simulink model "panda"  (R2022b)
settings: Solver=VariableStepAuto  StartTime=0.0  StopTime=10  EnableMultiTasking=on
values from neighbouring files (symbols this model uses):
  en = 1    [main_manipulator.m]
  q0 = [-pi/4 -3*pi/4]    [main_manipulator.m]
  q2 = [-0.785398163397 -0.78574787628 -0.786097014423 -0.786445577071 -0.786793563474 -0.787140972883 -0.787487804552 -0.787834057739 -0.788179731704 -0.788524825712 -0.78886933903 -0.789213270926 ... (6284 elements, 1x6284)]    [q2.mat]
  sr = 0.01    [main_manipulator.m]
  T = 1    [main_manipulator.m]
  w0 = 0.*[(q2(2)-q2(1))/(T/length(q2)) (q4(2)-q4(1))/(T/length(q4))]    [main_manipulator.m]
undefined symbols (not defined in the file or in its folder): Acceleration_1, Acceleration_2, Center_1, Center_2, magnitude, Pitch_1, Pitch_2, q4, Radius_1, Radius_2, Transformation_1, Transformation_2, tt, X, x_ee, Y, y_ee, Z
libraries: nesl_utility x15, sm_lib x14, simulink x14, slpidlib x4, franka_simulink_library x2, rllib x1
(part 1 of 2)
settings Model: Creator=Metti  LastModifiedBy=s2ajami
settings SolverCC: ZeroCrossControl=DisableAll
settings DataIOCC: LimitDataPoints=on  SaveFormat=Array  ReturnWorkspaceOutputs=off
settings OptimizationCC: ExpressionDepthLimit=2147483647  LifeSpan=inf
settings DebuggingCC: UnderspecifiedInitializationDetection=Classic  MergeDetectMultiDrivingBlocksExec=none  SolverPrmCheckMsg=warning  MultiTaskDSMMsg=warning  MultiTaskCondExecSysMsg=none  FcnCallInpInsideContextMsg=warning  UnconnectedInputMsg=warning  UnconnectedOutputMsg=warning  UnconnectedLineMsg=warning  StateNameClashWarn=warning  SFUnexpectedBacktrackingDiag=warning  SFNoUnconditionalDefaultTransitionDiag=warning  SFExecutionAtInitializationDiag=none  SFMachineParentedDataDiag=warning  ArithmeticOperatorsInVariantConditions=warning
settings HardwareCC: ProdBitPerPointer=32  ProdBitPerSizeT=32  ProdBitPerPtrDiffT=32  ProdLargestAtomicFloat=None  ProdIntDivRoundTo=Undefined  ProdEndianess=Unspecified  ProdWordSize=32  ProdHWDeviceType=32-bit Generic
settings ModelReferenceCC: EnableRefExpFcnMdlSchedulingChecks=on  PropagateSignalLabelsOutOfModel=off
settings SFSimCC: SimUseLocalCustomCode=off  CustomCodeUndefinedFunction=UseInterfaceOnly
settings RTWCC: RTWUseLocalCustomCode=off
settings CodeAppCC: StateflowObjectComments=on
settings GRTTargetCC: TargetLangStandard=C89/C90 (ANSI)
settings ConfigComp: CovMetricSettings=dw  CovSaveCumulativeToWorkspaceVar=on  CovSaveSingleToWorkspaceVar=on  CovExternalEMLEnable=off
settings SimscapeCC: SimscapeNormalizeSystem=off
settings ConfigurationSet: Description=SimMechanics 2G
settings ExplorerConfigSet: InternalSimMechanicsExplorerSettings="<ExplorerConfiguration><canonicalview>default</canonicalview><TilePanel><TileInfo><Tiles Columns=\"1\" Count=\"1\" Rows=\"1\"><Column Left=\"2\" Weight=\"1\"/><Column Left=\"539\"/><Row Top=\"2\" Weight=\"1\"/><Row Top=\"740\"/><Tile Height=\"1\" Width=\"1\" X=\"0\" Y=\"0\"/></Tiles></TileInfo><SceneInfo><SceneViewer><BGColor><R>0.60000002384185791</R><G>0.60000002384185791</G><B>0.60000002384185791</B></BGColor><Camera><Position><X>0.12540884528620469</X><Y>-2.4061754559467787</Y><Z>5.7088883074161094</Z></Position><Center><X>0.12540884528620469</X><Y>-2.4061754559467787</Y><Z>0</Z></Center><Up><X>0</X><Y>1</Y><Z>-0</Z></Up><Left>-3.8114177936930793</Left><Right>3.8114177936930793</Right><Bottom>-1.6453986206348663</Bottom><Top>1.6453986206348663</Top></Camera></SceneViewer></SceneInfo></TilePanel></ExplorerConfiguration>"

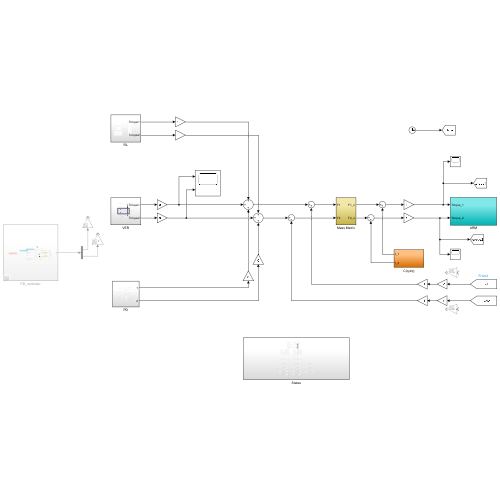
[thumbnail: Simulink's stored preview of the top-level diagram]
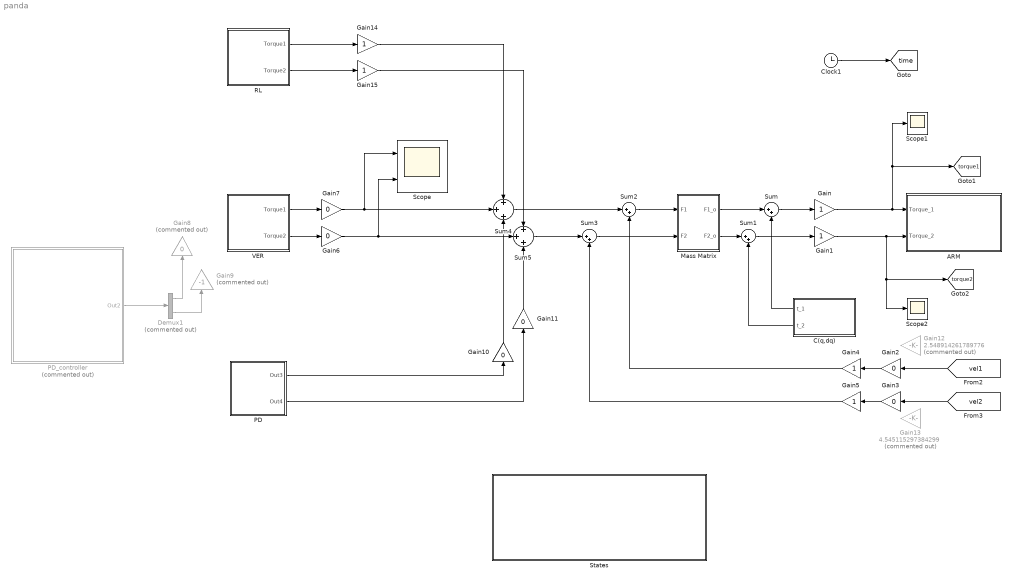
== system panda ==
  ARM : Subsystem
  C(q,dq) : Subsystem
  Clock1 : Clock
  Demux1 : Demux  Commented=on  Outputs=2
  Gain{,1,4..5,14..15} (6 alike) : Gain
  Gain{2..3,6..7,10..11} (6 alike) : Gain  Gain=0
  Gain12 : Gain  Commented=on  Gain=2.548914261789776
  Gain13 : Gain  Commented=on  Gain=4.545115297384299
  Gain8 : Gain  Commented=on  Gain=0
  Gain9 : Gain  Commented=on  Gain=-1
  Mass Matrix : Subsystem
  PD : Subsystem
  PD_controller : Subsystem  Commented=on
  RL : Subsystem
  Scope : Scope  NumInputPorts=2
  Scope1 : Scope
  Scope2 : Scope
  States : Subsystem
  Sum{,1..3} (4 alike) : Sum  Inputs=|++
  Sum4 : Sum  Inputs=+|+|+
  Sum5 : Sum  Inputs=+|+|+
  VER : Subsystem
  tag scope: time=global, torque1=global, torque2=global
  wires:
  Mass Matrix/1(F1_o) -> Sum/1
  Mass Matrix/2(F2_o) -> Sum1/1
  Sum1/1 -> Gain1/1
  [vel1] -> Gain2/1
  [vel2] -> Gain3/1
  Gain2/1 -> Gain4/1
  Gain3/1 -> Gain5/1
  Gain4/1 -> Sum2/2
  Gain5/1 -> Sum3/2
  VER/1(Torque1) -> Gain7/1
  Sum4/1 -> Sum2/1
  VER/2(Torque2) -> Gain6/1
  Sum5/1 -> Sum3/1
  Demux1/2 -> Gain9/1
  Demux1/1 -> Gain8/1
  PD_controller/1(Out2) -> Demux1/1
  Sum/1 -> Gain/1
  C(q,dq)/1(t_1) -> Sum/2
  C(q,dq)/2(t_2) -> Sum1/2
  Clock1/1 -> [time]
  Gain10/1 -> Sum4/3
  Gain7/1 -> Scope/1, Sum4/2
  Gain6/1 -> Scope/2, Sum5/2
  Gain11/1 -> Sum5/3
  Sum2/1 -> Mass Matrix/1(F1)
  Sum3/1 -> Mass Matrix/2(F2)
  Gain/1 -> Scope1/1, [torque1], ARM/1(Torque_1)
  Gain1/1 -> ARM/2(Torque_2), [torque2], Scope2/1
  PD/1(Out3) -> Gain10/1
  PD/2(Out4) -> Gain11/1
  RL/1(Torque1) -> Gain14/1
  RL/2(Torque2) -> Gain15/1
  Gain14/1 -> Sum4/1
  Gain15/1 -> Sum5/1

== system panda/ARM ==
  Torque_1 : Inport
  Torque_2 : Inport  Port=2
  G : Subsystem
  Scope : Scope
  Scope1 : Scope
  Subsystem : Subsystem
  Sum : Sum  Inputs=|++
  Sum1 : Sum  Inputs=|++
  tag scope: acc_ee=global, pos_ee=global, vel_ee=global
  wires:
  Torque_1/1 -> Scope/1, Sum1/1
  Torque_2/1 -> Sum/1
  G/1(t_1) -> Sum1/2
  G/2(t_2) -> Sum/2
  Sum1/1 -> Scope1/1, Subsystem/1(Torque_1)
  Sum/1 -> Subsystem/2(Torque_2)
  Subsystem/1(pos) -> [pos_ee]
  Subsystem/2(vel) -> [vel_ee]
  Subsystem/3(acc) -> [acc_ee]

== system panda/C(q,dq) ==
  Bias : Bias  Bias=pi/2  SaturateOnIntegerOverflow=off
  Demux : Demux  Outputs=2
  Gain{,1..2,12} (4 alike) : Gain  Gain=-1
  MATLAB Function1 : MATLAB Function  TreatAsAtomicUnit=on
  Mux1 : Mux  Inputs=6
  t_1 : Outport
  t_2 : Outport  Port=2
  wires:
  MATLAB Function1/1(y) -> Demux/1
  Demux/1 -> t_1/1
  Demux/2 -> Gain12/1
  Gain2/1 -> Mux1/6
  Gain1/1 -> Mux1/5
  [pos1] -> Bias/1
  Gain/1 -> Mux1/4
  [accel2] -> Gain2/1
  [vel2] -> Gain1/1
  Bias/1 -> Mux1/1
  [accel1] -> Mux1/3
  [vel1] -> Mux1/2
  [pos2] -> Gain/1
  Mux1/1 -> MATLAB Function1/1(u)
  Gain12/1 -> t_2/1

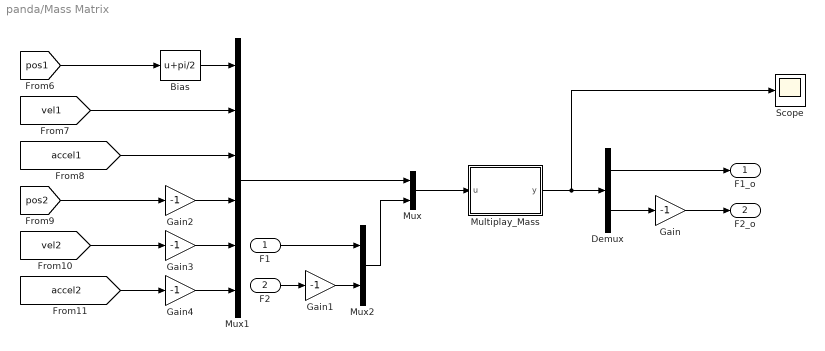
== system panda/Mass Matrix ==
  F1 : Inport
  F2 : Inport  Port=2
  Bias : Bias  Bias=pi/2  SaturateOnIntegerOverflow=off
  Demux : Demux  Outputs=2
  Gain{,1..4} (5 alike) : Gain  Gain=-1
  Multiplay_Mass : MATLAB Function  TreatAsAtomicUnit=on
  Mux : Mux  Inputs=2
  Mux1 : Mux  Inputs=6
  Mux2 : Mux  Inputs=2
  Scope : Scope
  F1_o : Outport
  F2_o : Outport  Port=2
  wires:
  Mux1/1 -> Mux/1
  Mux/1 -> Multiplay_Mass/1(u)
  F1/1 -> Mux2/1
  Gain1/1 -> Mux2/2
  Mux2/1 -> Mux/2
  Demux/1 -> F1_o/1
  Demux/2 -> Gain/1
  [accel2] -> Gain4/1
  [vel2] -> Gain3/1
  [pos1] -> Bias/1
  [pos2] -> Gain2/1
  Bias/1 -> Mux1/1
  [accel1] -> Mux1/3
  [vel1] -> Mux1/2
  Gain/1 -> F2_o/1
  F2/1 -> Gain1/1
  Gain2/1 -> Mux1/4
  Gain3/1 -> Mux1/5
  Gain4/1 -> Mux1/6
  Multiplay_Mass/1(y) -> Scope/1, Demux/1

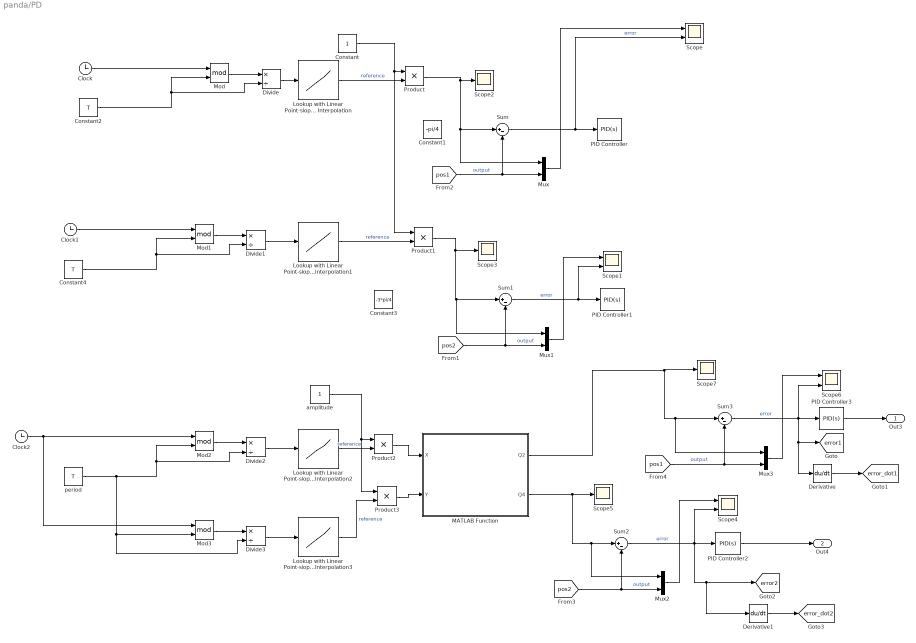
== system panda/PD ==
  Clock : Clock
  Clock1 : Clock
  Clock2 : Clock
  Constant : Constant
  Constant1 : Constant  Value=-pi/4
  Constant2 : Constant  Value=T
  Constant3 : Constant  Value=-3*pi/4
  Constant4 : Constant  Value=T
  Derivative : Derivative
  Derivative1 : Derivative
  Divide{,1..3} (4 alike) : Product  Inputs=*/
  Lookup with Linear Point-slope Interpolation : Lookup_n-D  NumberOfTableDimensions=1  BreakpointsForDimension1=linspace(0,1,length(q2))  Table=q2  InternalRulePriority=Speed  RndMeth=Simplest
  Lookup with Linear Point-slope Interpolation1 : Lookup_n-D  NumberOfTableDimensions=1  BreakpointsForDimension1=linspace(0,1,length(q4))  Table=q4  InternalRulePriority=Speed  RndMeth=Simplest
  Lookup with Linear Point-slope Interpolation2 : Lookup_n-D  NumberOfTableDimensions=1  BreakpointsForDimension1=linspace(0,1,length(x_ee))  Table=x_ee  InternalRulePriority=Speed  RndMeth=Simplest
  Lookup with Linear Point-slope Interpolation3 : Lookup_n-D  NumberOfTableDimensions=1  BreakpointsForDimension1=linspace(0,1,length(y_ee))  Table=y_ee  InternalRulePriority=Speed  RndMeth=Simplest
  MATLAB Function : MATLAB Function  TreatAsAtomicUnit=on
  Mod{,1..3} (4 alike) : Math  Operator=mod
  Mux{,1..3} (4 alike) : Mux  Inputs=2
  PID Controller{,1..3} (4 alike) : slpidlib/PID Controller  Controller=PID  Form=Parallel  TimeDomain=Continuous-time  UseExternalTs=off  SampleTime=-1  IntegratorMethod=Forward Euler  FilterMethod=Forward Euler  ControllerParametersSource=internal  P=150  I=0  UseKiTs=off  D=120  N=100  UseFilter=on  TunerSelectOption=Transfer Function Based (PID Tuner App)  InitialConditionSource=internal  InitialConditionForIntegrator=0  InitialConditionForFilter=0  DifferentiatorICPrevScaledInput=0  ExternalReset=none  TrackingMode=off  Kt=1  LimitOutput=off  SatLimitsSource=internal  UpperSaturationLimit=inf  LowerSaturationLimit=-inf  LinearizeAsGain=on  AntiWindupMode=none  Kb=1  LimitIntegrator=off  UpperIntegratorSaturationLimit=inf  LowerIntegratorSaturationLimit=-inf  POutMin=[]  POutMax=[]  IOutMin=[]  IOutMax=[]  DOutMin=[]  DOutMax=[]  NOutMin=[]  NOutMax=[]  SumOutMin=[]  SumOutMax=[]  SaturationOutMin=[]  SaturationOutMax=[]  PParamMin=[]  PParamMax=[]  IParamMin=[]  IParamMax=[]  DParamMin=[]  DParamMax=[]  NParamMin=[]  NParamMax=[]  KbParamMin=[]  KbParamMax=[]  KtParamMin=[]  KtParamMax=[]  KbOutMin=[]  KbOutMax=[]  KtOutMin=[]  KtOutMax=[]  IntegratorOutMin=[]  IntegratorOutMax=[]  FilterOutMin=[]  FilterOutMax=[]  SumI1OutMin=[]  SumI1OutMax=[]  SumI2OutMin=[]  SumI2OutMax=[]  SumI3OutMin=[]  SumI3OutMax=[]  SumI4OutMin=[]  SumI4OutMax=[]  SumDOutMin=[]  SumDOutMax=[]  DifferentiatorOutMin=[]  DifferentiatorOutMax=[]  FilterDiffOutCoefMin=[]  FilterDiffOutCoefMax=[]  ReciprocalOutMin=[]  ReciprocalOutMax=[]  SumDenOutMin=[]  SumDenOutMax=[]  SumNumOutMin=[]  SumNumOutMax=[]  DivideOutMin=[]  DivideOutMax=[]  UdiffTsProdOutMin=[]  UdiffTsProdOutMax=[]  NTsProdOutMin=[]  NTsProdOutMax=[]  UintegralTsProdOutMin=[]  UintegralTsProdOutMax=[]  UngainTsProdOutMin=[]  UngainTsProdOutMax=[]  ClampingZeroOutDataTypeStr=Inherit: Inherit via back propagation  ClampingZeroOutMin=[]  ClampingZeroOutMax=[]  FilterDenConstantOutDataTypeStr=Inherit: Inherit via back propagation  FilterDenConstantOutMin=[]  FilterDenConstantOutMax=[]  PCopyOutDataTypeStr=Inherit: Inherit via back propagation  PCopyOutMin=[]  PCopyOutMax=[]  NCopyOutDataTypeStr=Inherit: Inherit via back propagation  NCopyOutMin=[]  NCopyOutMax=[]  IntegratorContinuousStateAttributes=''  IntegratorStateMustResolveToSignalObject=off  IntegratorRTWStateStorageClass=Auto  FilterContinuousStateAttributes=''  FilterStateMustResolveToSignalObject=off  FilterRTWStateStorageClass=Auto  ParallelPVariant=InternalParameters  IdealPVariant=Disabled  IVariant=InternalParameters  DVariant=InternalParameters  IntegratorVariant=Continuous  SatVariant=Disabled  AWVariant=Passthrough  PCopyVariant=Disabled  TRVariant=Disabled  FdbkBlocksVariant=Forward  IdealPFdbkVariant=Disabled  SatFdbkVariant=Disabled  DerivativeFilterVariant=ContFilter  NVariant=InternalParameters  NCopyVariant=Disabled  FilterICVariant=InternalICsFilter  IntegratorICVariant=InternalICs  ExternalResetVariant=Disabled  TRSumVariant=Passthrough  SumFdbkVariant=Disabled  SumVariant=Sum_PID  TsampFilterVariant=InternalTs  TsampNgainVariant=Passthrough  TsampIntegralVariant=Passthrough  ExternalSaturationOutDataTypeStr=Inherit: Same as second input
  Product{,1..3} (4 alike) : Product
  Scope{,1,4,6} (4 alike) : Scope  NumInputPorts=2
  Scope{2..3,5,7} (4 alike) : Scope
  Sum{,1..3} (4 alike) : Sum  Inputs=|+-
  amplitude : Constant
  period : Constant  Value=T
  Out3 : Outport
  Out4 : Outport  Port=2
  tag scope: error1=global, error2=global, error_dot1=global, error_dot2=global
  wires:
  Sum/1 -> Scope/2, PID Controller/1  "error"
  [pos1] -> Sum/2, Mux/2  "output"
  Clock/1 -> Mod/1
  Mod/1 -> Divide/1
  Constant2/1 -> Divide/2, Mod/2
  Divide/1 -> Lookup with Linear Point-slope Interpolation/1
  Mux/1 -> Scope/1
  Mux1/1 -> Scope1/1
  Divide1/1 -> Lookup with Linear Point-slope Interpolation1/1
  Constant4/1 -> Mod1/2, Divide1/2
  Mod1/1 -> Divide1/1
  Clock1/1 -> Mod1/1
  [pos2] -> Mux1/2, Sum1/2  "output"
  Sum1/1 -> PID Controller1/1, Scope1/2  "error"
  Lookup with Linear Point-slope Interpolation/1 -> Product/2  "reference"
  Product/1 -> Mux/1, Sum/1, Scope2/1
  Constant/1 -> Product1/1, Product/1
  Lookup with Linear Point-slope Interpolation1/1 -> Product1/2  "reference"
  Clock2/1 -> Mod2/1, Mod3/1
  Mod2/1 -> Divide2/1
  period/1 -> Divide3/2, Mod3/2, Divide2/2, Mod2/2
  Divide2/1 -> Lookup with Linear Point-slope Interpolation2/1
  Divide3/1 -> Lookup with Linear Point-slope Interpolation3/1
  Mod3/1 -> Divide3/1
  Product1/1 -> Mux1/1, Sum1/1, Scope3/1
  Lookup with Linear Point-slope Interpolation2/1 -> Product2/2  "reference"
  Product2/1 -> MATLAB Function/1(X)
  Lookup with Linear Point-slope Interpolation3/1 -> Product3/2  "reference"
  Product3/1 -> MATLAB Function/2(Y)
  amplitude/1 -> Product3/1, Product2/1
  [pos2] -> Sum2/2, Mux2/2  "output"
  Mux2/1 -> Scope4/1
  Mux3/1 -> Scope6/1
  [pos1] -> Mux3/2, Sum3/2  "output"
  Sum3/1 -> Derivative/1, [error1], PID Controller3/1, Scope6/2  "error"
  MATLAB Function/1(Q2) -> Scope7/1, Mux3/1, Sum3/1
  PID Controller2/1 -> Out4/1
  PID Controller3/1 -> Out3/1
  Derivative/1 -> [error_dot1]
  Derivative1/1 -> [error_dot2]
  Sum2/1 -> Derivative1/1, [error2], Scope4/2, PID Controller2/1  "error"
  MATLAB Function/2(Q4) -> Mux2/1, Sum2/1, Scope5/1

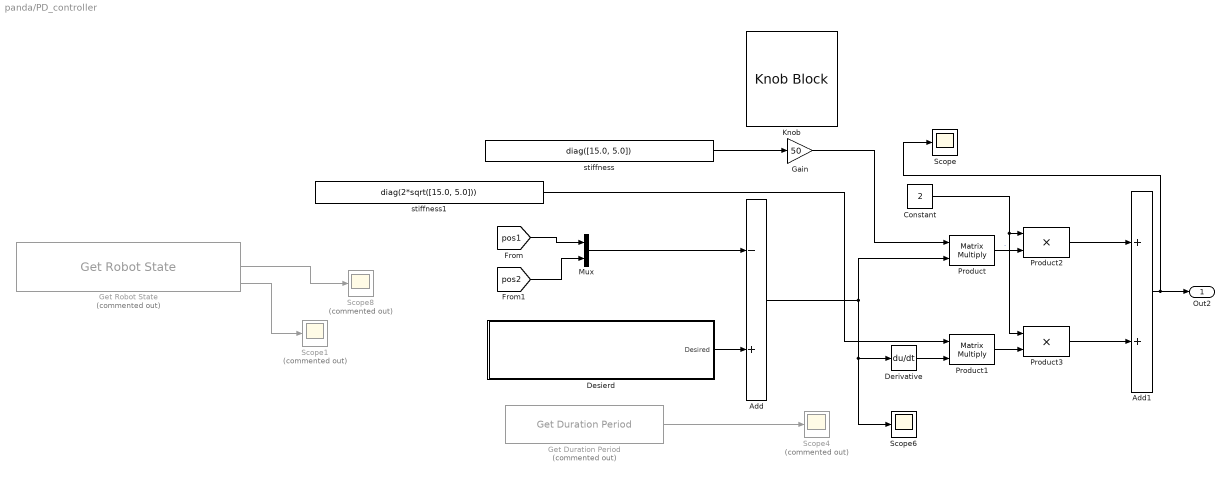
== system panda/PD_controller ==
  Add : Sum  Inputs=-+
  Add1 : Sum
  Constant : Constant  Value=2
  Derivative : Derivative
  Desierd : Subsystem
  Gain : Gain  Gain=50
  Get Duration Period : franka_simulink_library/Get Duration Period  Commented=on  robot_ip=robot_ip
  Get Robot State : franka_simulink_library/Get Robot State  Commented=on  robot_ip=robot_ip  signals_requested='q tau_J tau_J_d'
  Knob : KnobBlock  ScaleMax=50
  Mux : Mux  Inputs=2
  Product : Product  Multiplication=Matrix(*)
  Product1 : Product  Multiplication=Matrix(*)
  Product2 : Product
  Product3 : Product
  Scope : Scope
  Scope1 : Scope  Commented=on
  Scope4 : Scope  Commented=on
  Scope6 : Scope
  Scope8 : Scope  Commented=on
  stiffness : Constant  Value=diag([15.0, 5.0])
  stiffness1 : Constant  Value=diag(2*sqrt([15.0, 5.0]))  VectorParams1D=off
  Out2 : Outport  VectorParamsAs1DForOutWhenUnconnected=off
  wires:
  Product2/1 -> Add1/1
  Get Robot State/2 -> Scope8/1
  Get Duration Period/1 -> Scope4/1
  Add1/1 -> Out2/1, Scope/1
  Derivative/1 -> Product1/2
  Product3/1 -> Add1/2
  Add/1 -> Product/2, Scope6/1, Derivative/1
  Constant/1 -> Product3/1, Product2/1
  Product1/1 -> Product3/2
  Product/1 -> Product2/2  "."
  Desierd/1(Desired) -> Add/2
  stiffness1/1 -> Product1/1
  Get Robot State/3 -> Scope1/1
  stiffness/1 -> Gain/1
  Gain/1 -> Product/1
  [pos1] -> Mux/1
  [pos2] -> Mux/2
  Mux/1 -> Add/1

== system panda/RL ==
  Calculate Observation : Subsystem
  Calculate Reward : Subsystem
  Check If Done : Subsystem
  Demux : Demux  Outputs=2
  RL Agent : rllib/RL Agent  Agent=agent  ExternalActionAsInput=off  ProvideLastAction=off  ProvideCumRwd=on  TreatAsDirectFeedthrough=on  UseStrictObservationDataTypes=off
  Scope : Scope
  Torque1 : Outport
  Torque2 : Outport  Port=2
  wires:
  Calculate Observation/1(Out1) -> RL Agent/1
  Calculate Reward/1(Out1) -> RL Agent/2
  RL Agent/2 -> Scope/1
  Check If Done/1(Out1) -> RL Agent/3
  RL Agent/1 -> Demux/1
  Demux/1 -> Torque1/1
  Demux/2 -> Torque2/1

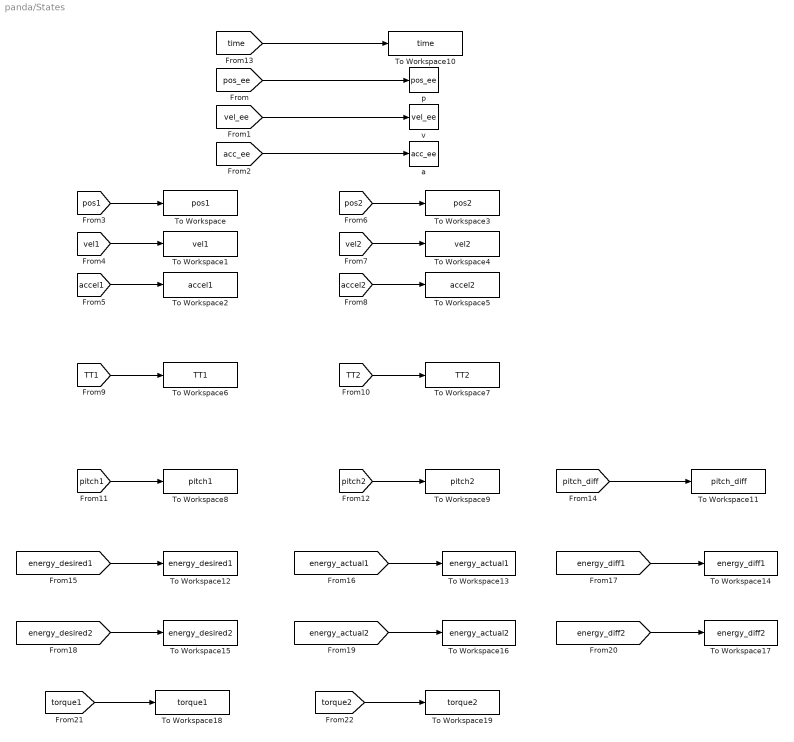
== system panda/States ==
  " a" : ToWorkspace  VariableName=acc_ee  SampleTime=sr
  " p" : ToWorkspace  VariableName=pos_ee  SampleTime=sr
  " v" : ToWorkspace  VariableName=vel_ee  SampleTime=sr
  To Workspace : ToWorkspace  VariableName=pos1  SampleTime=-1
  To Workspace1 : ToWorkspace  VariableName=vel1  SampleTime=-1
  To Workspace10 : ToWorkspace  VariableName=time  SampleTime=-1
  To Workspace11 : ToWorkspace  VariableName=pitch_diff  SampleTime=-1
  To Workspace12 : ToWorkspace  VariableName=energy_desired1  SampleTime=-1
  To Workspace13 : ToWorkspace  VariableName=energy_actual1  SampleTime=-1
  To Workspace14 : ToWorkspace  VariableName=energy_diff1  SampleTime=-1
  To Workspace15 : ToWorkspace  VariableName=energy_desired2  SampleTime=-1
  To Workspace16 : ToWorkspace  VariableName=energy_actual2  SampleTime=-1
  To Workspace17 : ToWorkspace  VariableName=energy_diff2  SampleTime=-1
  To Workspace18 : ToWorkspace  VariableName=torque1  SampleTime=-1
  To Workspace19 : ToWorkspace  VariableName=torque2  SampleTime=-1
  To Workspace2 : ToWorkspace  VariableName=accel1  SampleTime=-1
  To Workspace3 : ToWorkspace  VariableName=pos2  SampleTime=-1
  To Workspace4 : ToWorkspace  VariableName=vel2  SampleTime=-1
  To Workspace5 : ToWorkspace  VariableName=accel2  SampleTime=-1
  To Workspace6 : ToWorkspace  VariableName=TT1  SampleTime=-1
  To Workspace7 : ToWorkspace  VariableName=TT2  SampleTime=-1
  To Workspace8 : ToWorkspace  VariableName=pitch1  SampleTime=-1
  To Workspace9 : ToWorkspace  VariableName=pitch2  SampleTime=-1
  wires:
  [pos_ee] -> " p"/1
  [vel_ee] -> " v"/1
  [acc_ee] -> " a"/1
  [pos1] -> To Workspace/1
  [vel1] -> To Workspace1/1
  [accel1] -> To Workspace2/1
  [accel2] -> To Workspace5/1
  [vel2] -> To Workspace4/1
  [pos2] -> To Workspace3/1
  [TT1] -> To Workspace6/1
  [TT2] -> To Workspace7/1
  [pitch1] -> To Workspace8/1
  [pitch2] -> To Workspace9/1
  [time] -> To Workspace10/1
  [pitch_diff] -> To Workspace11/1
  [energy_desired1] -> To Workspace12/1
  [energy_actual1] -> To Workspace13/1
  [energy_diff1] -> To Workspace14/1
  [energy_diff2] -> To Workspace17/1
  [energy_actual2] -> To Workspace16/1
  [energy_desired2] -> To Workspace15/1
  [torque1] -> To Workspace18/1
  [torque2] -> To Workspace19/1

== system panda/VER ==
  note: synchronizer
  Cos : Trigonometry  Operator=cos
  Cos1 : Trigonometry  Operator=cos
  Dumble LC1 : Subsystem
  Dumble LC2 : Subsystem  Commented=on
  Gain : Gain  Gain=0
  Gain1 : Gain  Gain=-1
  Gain2 : Gain
  Gain3 : Gain
  Gain4 : Gain  Gain=3
  Joint LC : Subsystem
  Joint2 with lookup1 : Subsystem  Commented=on
  Joint2_without lookup : Subsystem  Commented=on
  Scope : Scope  NumInputPorts=2
  Scope3 : Scope
  Sum2 : Sum  Inputs=+|-
  Torque1 : Outport
  Torque2 : Outport  Port=2
  tag scope: pitch_diff=global
  wires:
  Gain/1 -> Dumble LC1/3(PC)
  Sum2/1 -> Gain4/1, [pitch_diff]
  [vel2] -> Dumble LC1/2(vel)
  Dumble LC1/2(Pitch) -> Scope/2, Cos/1
  Dumble LC1/1(Torque) -> Torque2/1
  [vel1] -> Joint LC/2(vel)
  Gain1/1 -> Joint LC/3(PC)
  Joint LC/1(Torque) -> Torque1/1
  Joint LC/2(Pitch) -> Cos1/1, Scope/1
  Cos/1 -> Gain2/1
  Cos1/1 -> Gain3/1, Scope3/1
  [pos1] -> Joint LC/1(pos)
  [pos2] -> Dumble LC1/1(pos)
  Gain2/1 -> Sum2/2
  Gain3/1 -> Sum2/1
  Gain4/1 -> Gain/1, Gain1/1

== system panda/ARM/G ==
  Bias : Bias  Bias=pi/2  SaturateOnIntegerOverflow=off
  Constant : Constant  Value=0.23
  Constant1 : Constant  Value=0.83
  Demux : Demux  Outputs=2
  Gain{,1..3} (4 alike) : Gain  Gain=-1
  Gain4 : Gain  Gain=0
  Gain5 : Gain  Gain=0
  MATLAB Function1 : MATLAB Function  TreatAsAtomicUnit=on
  Mux1 : Mux  Inputs=6
  Scope : Scope
  t_1 : Outport
  t_2 : Outport  Port=2
  wires:
  [accel1] -> Mux1/3
  [vel1] -> Mux1/2
  [pos1] -> Bias/1
  [accel2] -> Gain2/1
  [vel2] -> Gain1/1
  [pos2] -> Gain/1
  MATLAB Function1/1(y) -> Demux/1
  Mux1/1 -> MATLAB Function1/1(u)
  Demux/1 -> t_1/1
  Demux/2 -> Gain3/1
  Gain2/1 -> Mux1/6
  Gain1/1 -> Mux1/5
  Gain/1 -> Mux1/4
  Bias/1 -> Mux1/1
  MATLAB Function1/2(fs) -> Scope/1
  Gain3/1 -> t_2/1
  Constant/1 -> Gain4/1
  Constant1/1 -> Gain5/1
  Gain4/1 -> MATLAB Function1/2(bs1)
  Gain5/1 -> MATLAB Function1/3(bs2)

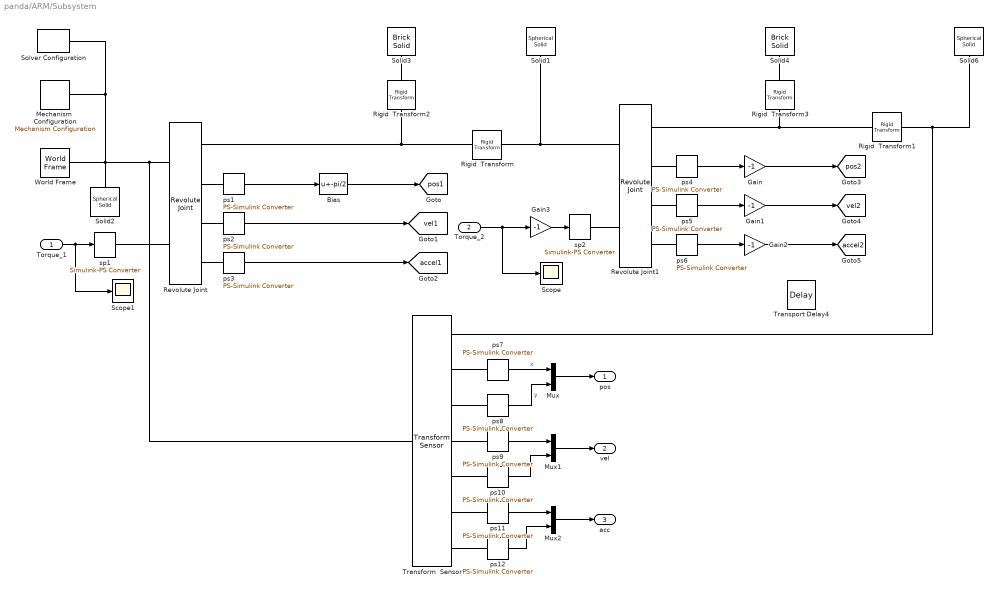
== system panda/ARM/Subsystem ==
  Torque_1 : Inport
  Torque_2 : Inport  Port=2
  Bias : Bias  Bias=-pi/2  SaturateOnIntegerOverflow=off
  Gain{,1..3} (4 alike) : Gain  Gain=-1
  Mechanism  Configuration : sm_lib/Utilities/Mechanism Configuration  UniformGravity=Constant  GravityVector=[0 -9.81 0]  GravityUnits=m/s^2  LinearizationDelta=0.0001  JointModeTransitionNonlinearIterations=2
  Mux : Mux  Inputs=2
  Mux1 : Mux  Inputs=2
  Mux2 : Mux  Inputs=2
  Revolute Joint : sm_lib/Joints/Revolute Joint  JointMode=Normal  SenseConstraintForce=off  SenseConstraintForceX=off  SenseConstraintForceY=off  SenseConstraintForceZ=off  SenseConstraintTorque=off  SenseConstraintTorqueX=off  SenseConstraintTorqueY=off  SenseConstraintTorqueZ=off  SenseTotalForce=off  SenseTotalForceX=off  SenseTotalForceY=off  SenseTotalForceZ=off  SenseTotalTorque=off  SenseTotalTorqueX=off  SenseTotalTorqueY=off  SenseTotalTorqueZ=off  CompositeWrenchDir=FollowerOnBase  CompositeWrenchFrame=BaseFrame  EquilibriumPosition=0  EquilibriumPositionUnits=deg  SpringStiffness=0  SpringStiffnessUnits=N*m/deg  DampingCoefficient=0  DampingCoefficientUnits=N*m/(deg/s)  TorqueActuationMode=InputTorque  MotionActuationMode=ComputedMotion  SensePosition=on  SenseVelocity=on  SenseAcceleration=on  SenseTorqueForce=off  SenseLowerLimitTorqueForce=off  SenseUpperLimitTorqueForce=off  LowerLimitSpecify=off  LowerLimitBound=-90  LowerLimitBoundUnits=deg  LowerLimitStiffness=1e4  LowerLimitStiffnessUnits=N*m/deg  LowerLimitDamping=10  LowerLimitDampingUnits=N*m/(deg/s)  LowerLimitTransitionRegionWidth=0.1  LowerLimitTransitionRegionWidthUnits=deg  UpperLimitSpecify=off  UpperLimitBound=90  UpperLimitBoundUnits=deg  UpperLimitStiffness=1e4  UpperLimitStiffnessUnits=N*m/deg  UpperLimitDamping=10  UpperLimitDampingUnits=N*m/(deg/s)  UpperLimitTransitionRegionWidth=0.1  UpperLimitTransitionRegionWidthUnits=deg  PositionTargetSpecify=on  PositionTargetPriority=High  PositionTargetValue=q0(1)+pi/2  PositionTargetValueUnits=rad  VelocityTargetSpecify=on  VelocityTargetPriority=High  VelocityTargetValue=w0(1)  VelocityTargetValueUnits=rad/s
  Revolute Joint1 : sm_lib/Joints/Revolute Joint  JointMode=Normal  SenseConstraintForce=off  SenseConstraintForceX=off  SenseConstraintForceY=off  SenseConstraintForceZ=off  SenseConstraintTorque=off  SenseConstraintTorqueX=off  SenseConstraintTorqueY=off  SenseConstraintTorqueZ=off  SenseTotalForce=off  SenseTotalForceX=off  SenseTotalForceY=off  SenseTotalForceZ=off  SenseTotalTorque=off  SenseTotalTorqueX=off  SenseTotalTorqueY=off  SenseTotalTorqueZ=off  CompositeWrenchDir=FollowerOnBase  CompositeWrenchFrame=BaseFrame  EquilibriumPosition=0  EquilibriumPositionUnits=deg  SpringStiffness=0  SpringStiffnessUnits=N*m/deg  DampingCoefficient=0  DampingCoefficientUnits=N*m/(deg/s)  TorqueActuationMode=InputTorque  MotionActuationMode=ComputedMotion  SensePosition=on  SenseVelocity=on  SenseAcceleration=on  SenseTorqueForce=off  SenseLowerLimitTorqueForce=off  SenseUpperLimitTorqueForce=off  LowerLimitSpecify=off  LowerLimitBound=-90  LowerLimitBoundUnits=deg  LowerLimitStiffness=1e4  LowerLimitStiffnessUnits=N*m/deg  LowerLimitDamping=10  LowerLimitDampingUnits=N*m/(deg/s)  LowerLimitTransitionRegionWidth=0.1  LowerLimitTransitionRegionWidthUnits=deg  UpperLimitSpecify=off  UpperLimitBound=90  UpperLimitBoundUnits=deg  UpperLimitStiffness=1e4  UpperLimitStiffnessUnits=N*m/deg  UpperLimitDamping=10  UpperLimitDampingUnits=N*m/(deg/s)  UpperLimitTransitionRegionWidth=0.1  UpperLimitTransitionRegionWidthUnits=deg  PositionTargetSpecify=on  PositionTargetPriority=High  PositionTargetValue=-q0(2)  PositionTargetValueUnits=rad  VelocityTargetSpecify=on  VelocityTargetPriority=High  VelocityTargetValue=-w0(2)  VelocityTargetValueUnits=rad/s
  Rigid  Transform : sm_lib/Frames and Transforms/Rigid Transform  TranslationMethod=StandardAxis  TranslationStandardOffset=1  TranslationLengthUnit=m  TranslationStandardAxis=+X  TranslationCartesianOffset=[0 0 0]  TranslationROffset=0  TranslationROffsetUnits=m  TranslationZOffset=0  TranslationZOffsetUnits=m  TranslationThetaOffset=0  TranslationThetaOffsetUnits=deg  RotationMethod=None  RotationAngleUnits=deg  RotationStandardAxis=+Z  RotationAngle=0  RotationArbitraryAxis=[0 0 1]  FollAlignAxisA=+X  BaseAlignAxisA=+Y  FollAlignAxisB=+Y  BaseAlignAxisB=+Z  RotationSequenceAxes=FollowerAxes  RotationSequence=XYX  RotationSequenceAngles=[0 0 0]  RotationSequenceAnglesUnits=deg  RotationMatrix=[1 0 0; 0 1 0; 0 0 1]  Quaternion=[1 0 0 0]
  Rigid  Transform1 : sm_lib/Frames and Transforms/Rigid Transform  TranslationMethod=StandardAxis  TranslationStandardOffset=1  TranslationLengthUnit=m  TranslationStandardAxis=+X  TranslationCartesianOffset=[0 0 0]  TranslationROffset=0  TranslationROffsetUnits=m  TranslationZOffset=0  TranslationZOffsetUnits=m  TranslationThetaOffset=0  TranslationThetaOffsetUnits=deg  RotationMethod=None  RotationAngleUnits=deg  RotationStandardAxis=+Z  RotationAngle=0  RotationArbitraryAxis=[0 0 1]  FollAlignAxisA=+X  BaseAlignAxisA=+Y  FollAlignAxisB=+Y  BaseAlignAxisB=+Z  RotationSequenceAxes=FollowerAxes  RotationSequence=XYX  RotationSequenceAngles=[0 0 0]  RotationSequenceAnglesUnits=deg  RotationMatrix=[1 0 0; 0 1 0; 0 0 1]  Quaternion=[1 0 0 0]
  Rigid  Transform2 : sm_lib/Frames and Transforms/Rigid Transform  TranslationMethod=StandardAxis  TranslationStandardOffset=1/2  TranslationLengthUnit=m  TranslationStandardAxis=+X  TranslationCartesianOffset=[0 0 0]  TranslationROffset=0  TranslationROffsetUnits=m  TranslationZOffset=0  TranslationZOffsetUnits=m  TranslationThetaOffset=0  TranslationThetaOffsetUnits=deg  RotationMethod=None  RotationAngleUnits=deg  RotationStandardAxis=+Z  RotationAngle=0  RotationArbitraryAxis=[0 0 1]  FollAlignAxisA=+X  BaseAlignAxisA=+Y  FollAlignAxisB=+Y  BaseAlignAxisB=+Z  RotationSequenceAxes=FollowerAxes  RotationSequence=XYX  RotationSequenceAngles=[0 0 0]  RotationSequenceAnglesUnits=deg  RotationMatrix=[1 0 0; 0 1 0; 0 0 1]  Quaternion=[1 0 0 0]
  Rigid  Transform3 : sm_lib/Frames and Transforms/Rigid Transform  TranslationMethod=StandardAxis  TranslationStandardOffset=1/2  TranslationLengthUnit=m  TranslationStandardAxis=+X  TranslationCartesianOffset=[0 0 0]  TranslationROffset=0  TranslationROffsetUnits=m  TranslationZOffset=0  TranslationZOffsetUnits=m  TranslationThetaOffset=0  TranslationThetaOffsetUnits=deg  RotationMethod=None  RotationAngleUnits=deg  RotationStandardAxis=+Z  RotationAngle=0  RotationArbitraryAxis=[0 0 1]  FollAlignAxisA=+X  BaseAlignAxisA=+Y  FollAlignAxisB=+Y  BaseAlignAxisB=+Z  RotationSequenceAxes=FollowerAxes  RotationSequence=XYX  RotationSequenceAngles=[0 0 0]  RotationSequenceAnglesUnits=deg  RotationMatrix=[1 0 0; 0 1 0; 0 0 1]  Quaternion=[1 0 0 0]
  Scope : Scope
  Scope1 : Scope
  Solid1 : sm_lib/Body Elements/Spherical Solid  GraphicAmbientColor=[0.15 0.15 0.15 1.0]  BasedOnType=Density  CenterOfMass=[0 0 0]  CenterOfMassUnits=m  GraphicDiffuseColor=[1.0 0.2 0.0]  Density=1000  DensityUnits=kg/(m^3)  DoExposeReferenceFrame=on  GraphicEmissiveColor=[0.0 0.0 0.0 1.0]  ExportEntireGeometry=off  SerializedExposedGeometries=<ExposedGeometries/>  SerializedFrames=<Frames/>  MarkerShape=Sphere  MarkerSize=10  GraphicType=FromGeometry  InertiaType=PointMass  Mass=0  MassUnits=kg  MomentsOfInertia=[1 1 1]  MomentsOfInertiaUnits=kg*m^2  GraphicOpacity=1.0  ProductsOfInertia=[0 0 0]  ProductsOfInertiaUnits=kg*m^2  GraphicShininess=75  GraphicSpecularColor=[0.5 0.5 0.5 1.0]  SphereRadius=0.1  SphereRadiusUnits=m  GraphicVisPropType=SimpleVisualProperties
  Solid2 : sm_lib/Body Elements/Spherical Solid  GraphicAmbientColor=[0.15 0.15 0.15 1.0]  BasedOnType=Density  CenterOfMass=[0 0 0]  CenterOfMassUnits=m  GraphicDiffuseColor=[0.0 0.0 1.0]  Density=1000  DensityUnits=kg/(m^3)  DoExposeReferenceFrame=on  GraphicEmissiveColor=[0.0 0.0 0.0 1.0]  ExportEntireGeometry=off  SerializedExposedGeometries=<ExposedGeometries/>  SerializedFrames=<Frames/>  MarkerShape=Sphere  MarkerSize=10  GraphicType=FromGeometry  InertiaType=PointMass  Mass=0  MassUnits=kg  MomentsOfInertia=[1 1 1]  MomentsOfInertiaUnits=kg*m^2  GraphicOpacity=1.0  ProductsOfInertia=[0 0 0]  ProductsOfInertiaUnits=kg*m^2  GraphicShininess=75  GraphicSpecularColor=[0.5 0.5 0.5 1.0]  SphereRadius=0.1  SphereRadiusUnits=m  GraphicVisPropType=SimpleVisualProperties
  Solid3 : sm_lib/Body Elements/Brick Solid  GraphicAmbientColor=[0.15 0.15 0.15 1.0]  BasedOnType=Mass  BrickDimensions=[1 .1 .1]  BrickDimensionUnits=m  CenterOfMass=[0 0 0]  CenterOfMassUnits=m  GraphicDiffuseColor=[0.8 0.8 0.0]  Density=1000  DensityUnits=kg/(m^3)  DoExposeReferenceFrame=on  GraphicEmissiveColor=[0.0 0.0 0.0 1.0]  ExportEntireGeometry=off  SerializedFrames=<Frames/>  MarkerShape=Sphere  MarkerSize=10  GraphicType=FromGeometry  InertiaType=CalculateFromGeometry  Mass=1  MassUnits=kg  MomentsOfInertia=[1 1 1]  MomentsOfInertiaUnits=kg*m^2  GraphicOpacity=1.0  ProductsOfInertia=[0 0 0]  ProductsOfInertiaUnits=kg*m^2  GraphicShininess=75  GraphicSpecularColor=[0.5 0.5 0.5 1.0]  GraphicVisPropType=SimpleVisualProperties
  Solid4 : sm_lib/Body Elements/Brick Solid  GraphicAmbientColor=[0.15 0.15 0.15 1.0]  BasedOnType=Mass  BrickDimensions=[1 .1 .1]  BrickDimensionUnits=m  CenterOfMass=[0 0 0]  CenterOfMassUnits=m  GraphicDiffuseColor=[0.8 0.8 0.0]  Density=1000  DensityUnits=kg/(m^3)  DoExposeReferenceFrame=on  GraphicEmissiveColor=[0.0 0.0 0.0 1.0]  ExportEntireGeometry=off  SerializedFrames=<Frames/>  MarkerShape=Sphere  MarkerSize=10  GraphicType=FromGeometry  InertiaType=CalculateFromGeometry  Mass=1  MassUnits=kg  MomentsOfInertia=[1 1 1]  MomentsOfInertiaUnits=kg*m^2  GraphicOpacity=1.0  ProductsOfInertia=[0 0 0]  ProductsOfInertiaUnits=kg*m^2  GraphicShininess=75  GraphicSpecularColor=[0.5 0.5 0.5 1.0]  GraphicVisPropType=SimpleVisualProperties
  Solid6 : sm_lib/Body Elements/Spherical Solid  GraphicAmbientColor=[0.15 0.15 0.15 1.0]  BasedOnType=Density  CenterOfMass=[0 0 0]  CenterOfMassUnits=m  GraphicDiffuseColor=[1.0 0.2 0.0]  Density=1000  DensityUnits=kg/(m^3)  DoExposeReferenceFrame=on  GraphicEmissiveColor=[0.0 0.0 0.0 1.0]  ExportEntireGeometry=off  SerializedExposedGeometries=<ExposedGeometries/>  SerializedFrames=<Frames/>  MarkerShape=Sphere  MarkerSize=10  GraphicType=FromGeometry  InertiaType=PointMass  Mass=0  MassUnits=kg  MomentsOfInertia=[1 1 1]  MomentsOfInertiaUnits=kg*m^2  GraphicOpacity=1.0  ProductsOfInertia=[0 0 0]  ProductsOfInertiaUnits=kg*m^2  GraphicShininess=75  GraphicSpecularColor=[0.5 0.5 0.5 1.0]  SphereRadius=0.1  SphereRadiusUnits=m  GraphicVisPropType=SimpleVisualProperties
  Solver Configuration : nesl_utility/Solver Configuration  PhysicalDomain=network_engine_domain  SubClassName=solver  LeftPortType=input  RightPortType=generic  Tones=[]  Harmonics=[]  SimulateNoise=off  Profile=off  UseLocalSampling=off  EnableSwitchedLinearOptims=on  FrequencyDomain=off  UseCCode=off  RelTol=0.001  AbsTol=1e-06  MinStep=1e-09  ToWorkspace=off  RevertToSquareIcSolve=off  NumHomotopyIterations=100  PhasorMode=off  PhasorModeNumHarmonics=1  ConsistencySolver=NEWTON_FTOL  IndexReductionMethod=DerivativeReplacement  DoDC=on  ResidualTolerance=1e-9  ConsistencyTolSource=GLOBAL  ConsistencyAbsTol=0.001  ConsistencyRelTol=0.001  ConsistencyTolFactor=0.001  UseLocalSolver=off  LocalSolverChoice=NE_BACKWARD_EULER_ADVANCER  ResolveIndetEquations=on  FunctionEvalNumThread=1  LocalSolverSampleTime=.001  DoFixedCost=off  MaxNonlinIter=3  MaxModeIter=2  ComputeImpulses=off  ImpulseIterations=2  LinearAlgebra=Sparse  LinearAlgebraNumThread=0  EquationFormulation=NE_TIME_EF  DelaysMemoryBudget=1024  AutomaticFiltering=on  FilteringTimeConstant=0.001  PartitionStorageMethod=AS_NEEDED  PartitionMemoryBudget=1024  PartitionMethod=FAST
  Transform  Sensor : sm_lib/Frames and Transforms/Transform Sensor  MeasurementFrame=World  SenseAngle=off  SenseAxis=off  SenseQ=off  SenseR=off  SenseRotationSequence=off  RotationSequence=XYX  SenseOmegaX=off  SenseOmegaY=off  SenseOmegaZ=off  SenseQDot=off  SenseRDot=off  SenseAlphaX=off  SenseAlphaY=off  SenseAlphaZ=off  SenseQDDot=off  SenseRDDot=off  SenseX=on  SenseY=on  SenseZ=off  SenseRad=off  SenseAzim=off  SenseDist=off  SenseInc=off  SenseXDot=on  SenseYDot=on  SenseZDot=off  SenseRadDot=off  SenseAzimDot=off  SenseDistDot=off  SenseIncDot=off  SenseXDDot=on  SenseYDDot=on  SenseZDDot=off  SenseRadDDot=off  SenseAzimDDot=off  SenseDistDDot=off  SenseIncDDot=off
  Transport Delay4 : TransportDelay  DelayTime=0.001
  World Frame : sm_lib/Frames and Transforms/World Frame
  ps{1..12} (12 alike) : nesl_utility/PS-Simulink Converter  PhysicalDomain=network_engine_domain  SubClassName=ps_output  LeftPortType=input  RightPortType=output  PseudoPeriodic=off  Frequencies=[]  VectorFormat=1-D array  Unit=1  AffineConversion=off
  sp1 : nesl_utility/Simulink-PS Converter  PhysicalDomain=network_engine_domain  SubClassName=ps_input  LeftPortType=input  RightPortType=output  PseudoPeriodic=off  Frequencies=[]  NoiseDistribution=none  NoiseParameters=[]  Unit=1  AffineConversion=off  FilteringAndDerivatives=zero  SimscapeFilterOrder=1  InputFilterTimeConstant=.001  UdotUserProvided=[]
  sp2 : nesl_utility/Simulink-PS Converter  PhysicalDomain=network_engine_domain  SubClassName=ps_input  LeftPortType=input  RightPortType=output  PseudoPeriodic=off  Frequencies=[]  NoiseDistribution=none  NoiseParameters=[]  Unit=1  AffineConversion=off  FilteringAndDerivatives=zero  SimscapeFilterOrder=1  InputFilterTimeConstant=.001  UdotUserProvided=[]
  pos : Outport
  vel : Outport  Port=2
  acc : Outport  Port=3
  tag scope: accel1=global, accel2=global, pos1=global, pos2=global, vel1=global, vel2=global
  wires:
  ps5/1 -> Gain1/1
  ps12/1 -> Mux2/2
  ps6/1 -> Gain2/1
  Mux/1 -> pos/1
  ps4/1 -> Gain/1
  ps7/1 -> Mux/1  "x"
  ps8/1 -> Mux/2  "y"
  Mux1/1 -> vel/1
  ps9/1 -> Mux1/1
  ps11/1 -> Mux2/1
  ps10/1 -> Mux1/2
  Mux2/1 -> acc/1
  Torque_2/1 -> Gain3/1, Scope/1
  Torque_1/1 -> Scope1/1, sp1/1
  Gain3/1 -> sp2/1
  ps1/1 -> Bias/1
  Gain/1 -> [pos2]
  Gain1/1 -> [vel2]
  Gain2/1 -> [accel2]
  Bias/1 -> [pos1]
  ps2/1 -> [vel1]
  ps3/1 -> [accel1]
  connections:
  ps2/LConn1 -- Revolute Joint/RConn3
  Revolute Joint1/LConn1 -- Solid1/RConn1 -- Rigid  Transform/RConn1
  Solid4/RConn1 -- Rigid  Transform3/RConn1
  Transform  Sensor/RConn7 -- ps12/LConn1
  World Frame/RConn1 -- Transform  Sensor/LConn1 -- Revolute Joint/LConn1 -- Mechanism  Configuration/RConn1 -- Solver Configuration/RConn1 -- Solid2/RConn1
  ps6/LConn1 -- Revolute Joint1/RConn4
  Rigid  Transform/LConn1 -- Revolute Joint/RConn1 -- Rigid  Transform2/LConn1
  sp2/RConn1 -- Revolute Joint1/LConn2
  Revolute Joint1/RConn3 -- ps5/LConn1
  sp1/RConn1 -- Revolute Joint/LConn2
  ps7/LConn1 -- Transform  Sensor/RConn2
  Transform  Sensor/RConn4 -- ps9/LConn1
  Rigid  Transform2/RConn1 -- Solid3/RConn1
  ps1/LConn1 -- Revolute Joint/RConn2
  Transform  Sensor/RConn1 -- Solid6/RConn1 -- Rigid  Transform1/RConn1
  Rigid  Transform3/LConn1 -- Revolute Joint1/RConn1 -- Rigid  Transform1/LConn1
  ps3/LConn1 -- Revolute Joint/RConn4
  Transform  Sensor/RConn5 -- ps10/LConn1
  Transform  Sensor/RConn3 -- ps8/LConn1
  Transform  Sensor/RConn6 -- ps11/LConn1
  ps4/LConn1 -- Revolute Joint1/RConn2

== system panda/PD_controller/Desierd ==
  Mux : Mux  Inputs=2
  Sine Wave1 : Sin  Amplitude=0  Bias=-pi/4  SampleTime=0
  Sine Wave3 : Sin  Amplitude=0  Bias=-3 * pi/4  SampleTime=0
  Desired : Outport  VectorParamsAs1DForOutWhenUnconnected=off
  wires:
  Sine Wave3/1 -> Mux/2
  Mux/1 -> Desired/1
  Sine Wave1/1 -> Mux/1

== system panda/RL/Calculate Observation ==
  Mux : Mux  Inputs=8
  Rate Transition : RateTransition
  Out1 : Outport
  wires:
  Mux/1 -> Rate Transition/1
  [pos1] -> Mux/1
  [vel1] -> Mux/2
  Rate Transition/1 -> Out1/1
  [error1] -> Mux/3
  [error_dot1] -> Mux/4
  [pos2] -> Mux/5
  [vel2] -> Mux/6
  [error2] -> Mux/7
  [error_dot2] -> Mux/8

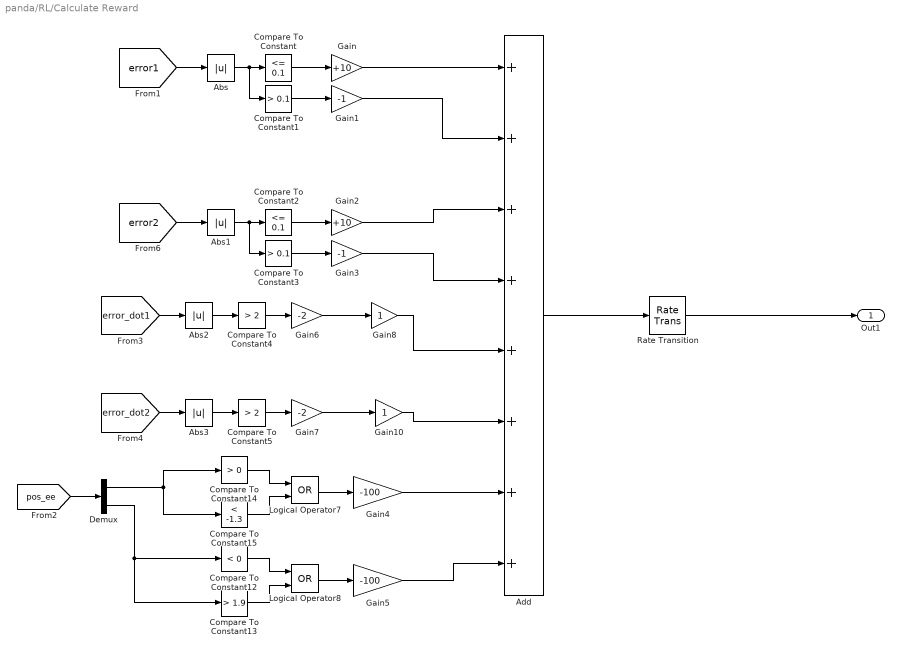
== system panda/RL/Calculate Reward ==
  Abs{,1..3} (4 alike) : Abs  SaturateOnIntegerOverflow=off
  Add : Sum  Inputs=++++++++
  Compare To Constant : simulink/Logic and Bit Operations/Compare To Constant  relop=<=  const=0.1  OutDataTypeStr=boolean
  Compare To Constant1 : simulink/Logic and Bit Operations/Compare To Constant  relop=>  const=0.1  OutDataTypeStr=boolean
  Compare To Constant12 : simulink/Logic and Bit Operations/Compare To Constant  relop=<  const=0  OutDataTypeStr=boolean
  Compare To Constant13 : simulink/Logic and Bit Operations/Compare To Constant  relop=>  const=1.9  OutDataTypeStr=boolean
  Compare To Constant14 : simulink/Logic and Bit Operations/Compare To Constant  relop=>  const=0  OutDataTypeStr=boolean
  Compare To Constant15 : simulink/Logic and Bit Operations/Compare To Constant  relop=<  const=-1.3  OutDataTypeStr=boolean
  Compare To Constant2 : simulink/Logic and Bit Operations/Compare To Constant  relop=<=  const=0.1  OutDataTypeStr=boolean
  Compare To Constant3 : simulink/Logic and Bit Operations/Compare To Constant  relop=>  const=0.1  OutDataTypeStr=boolean
  Compare To Constant4 : simulink/Logic and Bit Operations/Compare To Constant  relop=>  const=2  OutDataTypeStr=boolean
  Compare To Constant5 : simulink/Logic and Bit Operations/Compare To Constant  relop=>  const=2  OutDataTypeStr=boolean
  Demux : Demux  Outputs=2
  Gain : Gain  Gain=+10
  Gain1 : Gain  Gain=-1
  Gain10 : Gain
  Gain2 : Gain  Gain=+10
  Gain3 : Gain  Gain=-1
  Gain4 : Gain  Gain=-100
  Gain5 : Gain  Gain=-100
  Gain6 : Gain  Gain=-2
  Gain7 : Gain  Gain=-2
  Gain8 : Gain
  Logical Operator7 : Logic  Operator=OR  AllPortsSameDT=off  OutDataTypeStr=boolean
  Logical Operator8 : Logic  Operator=OR  AllPortsSameDT=off  OutDataTypeStr=boolean
  Rate Transition : RateTransition
  Out1 : Outport
  wires:
  Add/1 -> Rate Transition/1
  Rate Transition/1 -> Out1/1
  [error1] -> Abs/1
  Abs/1 -> Compare To Constant1/1, Compare To Constant/1
  Compare To Constant/1 -> Gain/1
  Gain/1 -> Add/1
  Compare To Constant1/1 -> Gain1/1
  Gain1/1 -> Add/2
  Compare To Constant3/1 -> Gain3/1
  Compare To Constant2/1 -> Gain2/1
  Abs1/1 -> Compare To Constant2/1, Compare To Constant3/1
  [error2] -> Abs1/1
  [pos_ee] -> Demux/1
  Compare To Constant12/1 -> Logical Operator8/1
  Demux/2 -> Compare To Constant13/1, Compare To Constant12/1
  Demux/1 -> Compare To Constant15/1, Compare To Constant14/1
  Compare To Constant14/1 -> Logical Operator7/1
  Compare To Constant13/1 -> Logical Operator8/2
  Compare To Constant15/1 -> Logical Operator7/2
  Logical Operator7/1 -> Gain4/1
  Logical Operator8/1 -> Gain5/1
  Gain4/1 -> Add/7
  Gain5/1 -> Add/8
  [error_dot2] -> Abs3/1
  [error_dot1] -> Abs2/1
  Abs2/1 -> Compare To Constant4/1
  Compare To Constant4/1 -> Gain6/1
  Gain6/1 -> Gain8/1
  Abs3/1 -> Compare To Constant5/1
  Compare To Constant5/1 -> Gain7/1
  Gain7/1 -> Gain10/1
  Gain2/1 -> Add/3
  Gain3/1 -> Add/4
  Gain10/1 -> Add/6
  Gain8/1 -> Add/5

== system panda/RL/Check If Done ==
  Compare To Constant12 : simulink/Logic and Bit Operations/Compare To Constant  relop=<  const=0  OutDataTypeStr=boolean
  Compare To Constant13 : simulink/Logic and Bit Operations/Compare To Constant  relop=>  const=1.9  OutDataTypeStr=boolean
  Compare To Constant14 : simulink/Logic and Bit Operations/Compare To Constant  relop=>  const=0  OutDataTypeStr=boolean
  Compare To Constant15 : simulink/Logic and Bit Operations/Compare To Constant  relop=<  const=-1.3  OutDataTypeStr=boolean
  Demux : Demux  Outputs=2
  Logical Operator : Logic  Operator=OR  AllPortsSameDT=off  OutDataTypeStr=boolean
  Logical Operator7 : Logic  Operator=OR  AllPortsSameDT=off  OutDataTypeStr=boolean
  Logical Operator8 : Logic  Operator=OR  AllPortsSameDT=off  OutDataTypeStr=boolean
  Out1 : Outport
  wires:
  Compare To Constant12/1 -> Logical Operator8/1
  Compare To Constant13/1 -> Logical Operator8/2
  Compare To Constant15/1 -> Logical Operator7/2
  Compare To Constant14/1 -> Logical Operator7/1
  [pos_ee] -> Demux/1
  Demux/1 -> Compare To Constant15/1, Compare To Constant14/1
  Demux/2 -> Compare To Constant13/1, Compare To Constant12/1
  Logical Operator/1 -> Out1/1
  Logical Operator7/1 -> Logical Operator/1
  Logical Operator8/1 -> Logical Operator/2

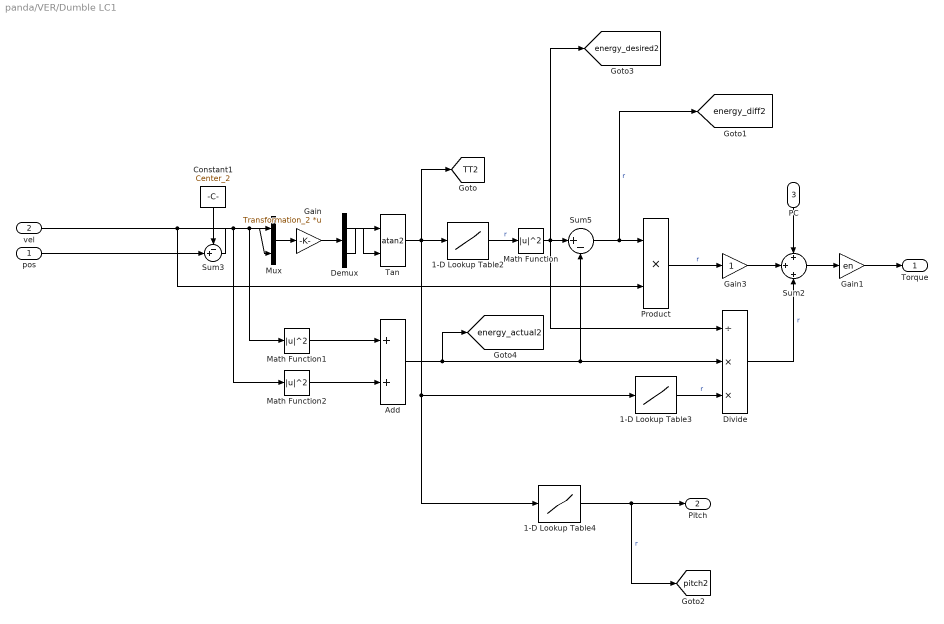
== system panda/VER/Dumble LC1 ==
  pos : Inport
  vel : Inport  Port=2
  PC : Inport  Port=3
  1-D Lookup Table2 : Lookup_n-D  NumberOfTableDimensions=1  BreakpointsForDimension1=tt  Table=Radius_2  InternalRulePriority=Speed  RndMeth=Simplest
  1-D Lookup Table3 : Lookup_n-D  NumberOfTableDimensions=1  BreakpointsForDimension1=tt  Table=Acceleration_2  InternalRulePriority=Speed  RndMeth=Simplest
  1-D Lookup Table4 : Lookup_n-D  NumberOfTableDimensions=1  BreakpointsForDimension1=tt  Table=Pitch_2  InternalRulePriority=Speed  RndMeth=Simplest
  Add : Sum
  Constant1 : Constant  Value=Center_2
  Demux : Demux  Outputs=2
  Divide : Product  Inputs=/**
  Gain : Gain  Gain=Transformation_2  Multiplication=Matrix(K*u)
  Gain1 : Gain  Gain=en
  Gain3 : Gain
  Math Function : Math  Operator=magnitude^2
  Math Function1 : Math  Operator=magnitude^2
  Math Function2 : Math  Operator=magnitude^2
  Mux : Mux  Inputs=2
  Product : Product
  Sum2 : Sum  Inputs=+|+|+
  Sum3 : Sum  Inputs=-+|
  Sum5 : Sum  Inputs=|+-
  Tan : Trigonometry  Operator=atan2
  Torque : Outport
  Pitch : Outport  Port=2
  tag scope: TT2=global, energy_actual2=global, energy_desired2=global, energy_diff2=global, pitch2=global
  wires:
  Gain1/1 -> Torque/1
  Demux/2 -> Tan/1
  Demux/1 -> Tan/2
  Mux/1 -> Gain/1
  Gain/1 -> Demux/1
  Divide/1 -> Sum2/3  "r"
  1-D Lookup Table3/1 -> Divide/3  "r"
  Add/1 -> [energy_actual2], Divide/2, Sum5/2
  PC/1 -> Sum2/1
  Gain3/1 -> Sum2/2
  1-D Lookup Table2/1 -> Math Function/1  "r"
  Constant1/1 -> Sum3/1
  Sum3/1 -> Math Function1/1, Mux/1
  Math Function1/1 -> Add/1
  Math Function2/1 -> Add/2
  pos/1 -> Sum3/2
  vel/1 -> Math Function2/1, Mux/2, Product/2
  Product/1 -> Gain3/1  "r"
  Sum2/1 -> Gain1/1
  Tan/1 -> [TT2], 1-D Lookup Table2/1, 1-D Lookup Table3/1, 1-D Lookup Table4/1
  1-D Lookup Table4/1 -> [pitch2], Pitch/1  "r"
  Sum5/1 -> Product/1, [energy_diff2]  "r"
  Math Function/1 -> [energy_desired2], Sum5/1, Divide/1

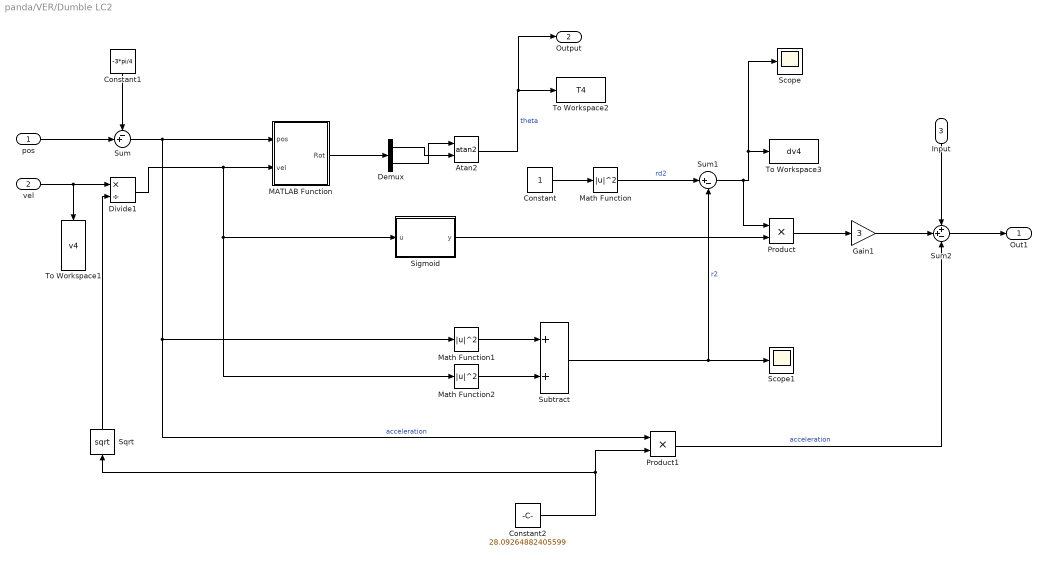
== system panda/VER/Dumble LC2 ==
  pos : Inport
  vel : Inport  Port=2
  Input : Inport  Port=3
  Atan2 : Trigonometry  Operator=atan2
  Constant : Constant
  Constant1 : Constant  Value=-3*pi/4
  Constant2 : Constant  Value=28.09264882405599
  Demux : Demux  Outputs=2
  Divide1 : Product  Inputs=*/
  Gain1 : Gain  Gain=3
  MATLAB Function : MATLAB Function  TreatAsAtomicUnit=on
  Math Function : Math  Operator=magnitude^2  SignedPower=on
  Math Function1 : Math  Operator=magnitude^2  SignedPower=on
  Math Function2 : Math  Operator=magnitude^2  SignedPower=on
  Product : Product
  Product1 : Product
  Scope : Scope
  Scope1 : Scope
  Sigmoid : MATLAB Function  TreatAsAtomicUnit=on
  Sqrt : Sqrt
  Subtract : Sum
  Sum : Sum  Inputs=-+|
  Sum1 : Sum  Inputs=|+-
  Sum2 : Sum  Inputs=++-
  To Workspace1 : ToWorkspace  VariableName=v4  SampleTime=-1
  To Workspace2 : ToWorkspace  VariableName=T4  SampleTime=-1
  To Workspace3 : ToWorkspace  VariableName=dv4  SampleTime=-1
  Out1 : Outport  VectorParamsAs1DForOutWhenUnconnected=off
  Output : Outport  Port=2  VectorParamsAs1DForOutWhenUnconnected=off
  wires:
  Sqrt/1 -> Divide1/2
  Divide1/1 -> MATLAB Function/2(vel), Sigmoid/1(u), Math Function2/1
  Constant2/1 -> Product1/2, Sqrt/1
  Product1/1 -> Sum2/3  "acceleration"
  Math Function2/1 -> Subtract/2
  Constant1/1 -> Sum/1
  Sigmoid/1(y) -> Product/2
  Sum/1 -> MATLAB Function/1(pos), Math Function1/1, Product1/1  "acceleration"
  Sum1/1 -> Product/1, To Workspace3/1, Scope/1
  Subtract/1 -> Scope1/1, Sum1/2  "r2"
  Sum2/1 -> Out1/1
  Atan2/1 -> To Workspace2/1, Output/1  "theta"
  pos/1 -> Sum/2
  Math Function/1 -> Sum1/1  "rd2"
  MATLAB Function/1(Rot) -> Demux/1
  Gain1/1 -> Sum2/2
  Demux/2 -> Atan2/1
  vel/1 -> Divide1/1, To Workspace1/1
  Demux/1 -> Atan2/2
  Input/1 -> Sum2/1
  Math Function1/1 -> Subtract/1
  Constant/1 -> Math Function/1
  Product/1 -> Gain1/1

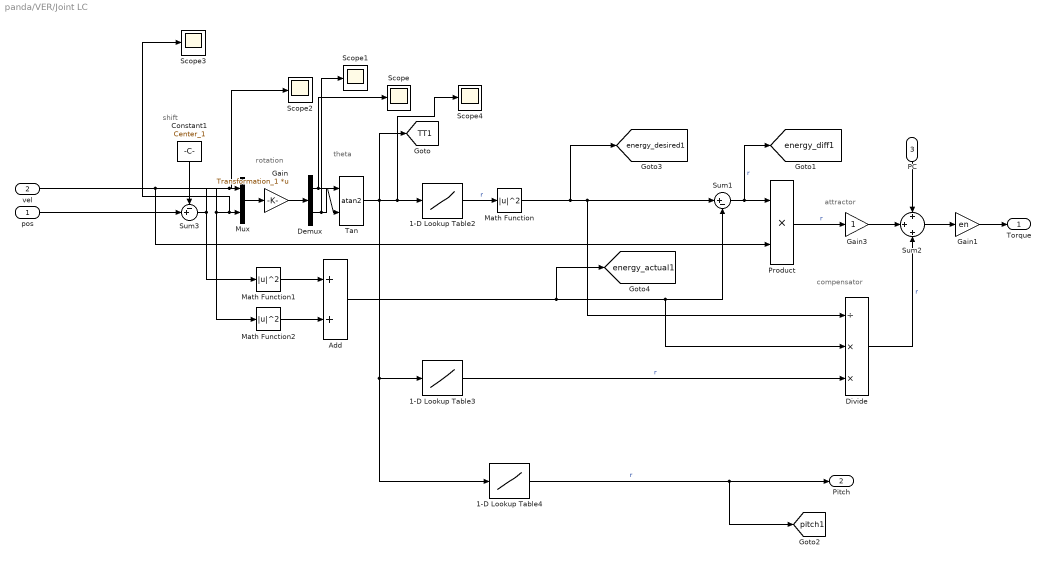
== system panda/VER/Joint LC ==
  note: compensator
  note: attractor
  note: theta
  note: rotation
  note: shift
  pos : Inport
  vel : Inport  Port=2
  PC : Inport  Port=3
  1-D Lookup Table2 : Lookup_n-D  NumberOfTableDimensions=1  BreakpointsForDimension1=tt  Table=Radius_1  InternalRulePriority=Speed  RndMeth=Simplest
  1-D Lookup Table3 : Lookup_n-D  NumberOfTableDimensions=1  BreakpointsForDimension1=tt  Table=Acceleration_1  InternalRulePriority=Speed  RndMeth=Simplest
  1-D Lookup Table4 : Lookup_n-D  NumberOfTableDimensions=1  BreakpointsForDimension1=tt  Table=Pitch_1  InternalRulePriority=Speed  RndMeth=Simplest
  Add : Sum
  Constant1 : Constant  Value=Center_1
  Demux : Demux  Outputs=2
  Divide : Product  Inputs=/**
  Gain : Gain  Gain=Transformation_1  Multiplication=Matrix(K*u)
  Gain1 : Gain  Gain=en
  Gain3 : Gain
  Math Function : Math  Operator=magnitude^2
  Math Function1 : Math  Operator=magnitude^2
  Math Function2 : Math  Operator=magnitude^2
  Mux : Mux  Inputs=2
  Product : Product
  Scope{,1..4} (5 alike) : Scope
  Sum1 : Sum  Inputs=|+-
  Sum2 : Sum  Inputs=+|+|+
  Sum3 : Sum  Inputs=-+|
  Tan : Trigonometry  Operator=atan2
  Torque : Outport
  Pitch : Outport  Port=2
  tag scope: TT1=global, energy_actual1=global, energy_desired1=global, energy_diff1=global, pitch1=global
  wires:
  Add/1 -> [energy_actual1], Sum1/2, Divide/2
  Sum2/1 -> Gain1/1
  1-D Lookup Table4/1 -> [pitch1], Pitch/1  "r"
  Product/1 -> Gain3/1  "r"
  vel/1 -> Product/2, Math Function2/1, Scope3/1, Mux/2
  pos/1 -> Sum3/2
  Math Function2/1 -> Add/2
  Math Function1/1 -> Add/1
  Sum1/1 -> [energy_diff1], Product/1  "r"
  Sum3/1 -> Math Function1/1, Scope2/1, Mux/1
  Constant1/1 -> Sum3/1
  Gain3/1 -> Sum2/2
  PC/1 -> Sum2/1
  1-D Lookup Table3/1 -> Divide/3  "r"
  Divide/1 -> Sum2/3  "r"
  Math Function/1 -> [energy_desired1], Sum1/1, Divide/1
  Mux/1 -> Gain/1
  Gain/1 -> Demux/1
  Tan/1 -> [TT1], 1-D Lookup Table4/1, 1-D Lookup Table3/1, Scope4/1, 1-D Lookup Table2/1
  Gain1/1 -> Torque/1
  1-D Lookup Table2/1 -> Math Function/1  "r"
  Demux/1 -> Scope/1, Tan/2
  Demux/2 -> Scope1/1, Tan/1

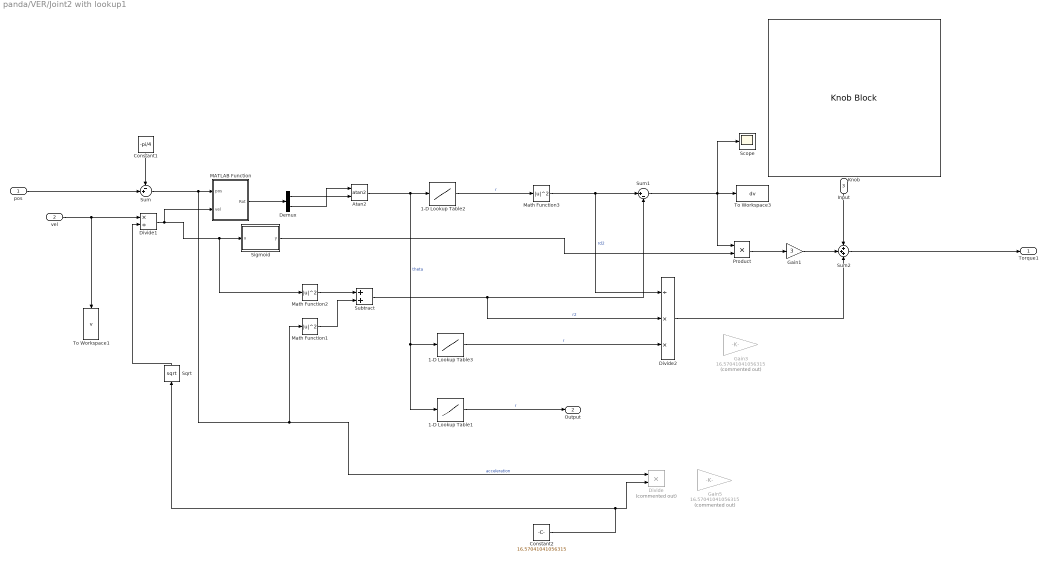
== system panda/VER/Joint2 with lookup1 ==
  pos : Inport
  vel : Inport  Port=2
  Input : Inport  Port=3
  1-D Lookup Table1 : Lookup_n-D  NumberOfTableDimensions=1  BreakpointsForDimension1=tt  Table=Pitch_1  InternalRulePriority=Speed  RndMeth=Simplest
  1-D Lookup Table2 : Lookup_n-D  NumberOfTableDimensions=1  BreakpointsForDimension1=tt  Table=Radius_1  InternalRulePriority=Speed  RndMeth=Simplest
  1-D Lookup Table3 : Lookup_n-D  NumberOfTableDimensions=1  BreakpointsForDimension1=tt  Table=Acceleration_1  InternalRulePriority=Speed  RndMeth=Simplest
  Atan2 : Trigonometry  Operator=atan2
  Constant1 : Constant  Value=-pi/4
  Constant2 : Constant  Value=16.57041041056315
  Demux : Demux  Outputs=2
  Divide : Product  Commented=on  Inputs=**
  Divide1 : Product  Inputs=*/
  Divide2 : Product  Inputs=/**
  Gain1 : Gain  Gain=3
  Gain3 : Gain  Commented=on  Gain=16.57041041056315
  Gain5 : Gain  Commented=on  Gain=16.57041041056315
  Knob : KnobBlock  ScaleMax=3  TickInterval=0.10000000000000001
  MATLAB Function : MATLAB Function  TreatAsAtomicUnit=on
  Math Function1 : Math  Operator=magnitude^2  SignedPower=on
  Math Function2 : Math  Operator=magnitude^2  SignedPower=on
  Math Function3 : Math  Operator=magnitude^2  SignedPower=on
  Product : Product
  Scope : Scope
  Sigmoid : MATLAB Function  TreatAsAtomicUnit=on
  Sqrt : Sqrt
  Subtract : Sum
  Sum : Sum  Inputs=-+|
  Sum1 : Sum  Inputs=|+-
  Sum2 : Sum  Inputs=+++
  To Workspace1 : ToWorkspace  VariableName=v  SampleTime=-1
  To Workspace3 : ToWorkspace  VariableName=dv  SampleTime=-1
  Torque1 : Outport  VectorParamsAs1DForOutWhenUnconnected=off
  Output : Outport  Port=2
  wires:
  1-D Lookup Table1/1 -> Output/1  "r"
  Divide2/1 -> Sum2/3
  Math Function1/1 -> Subtract/2
  Math Function2/1 -> Subtract/1
  Subtract/1 -> Divide2/2, Sum1/2  "r2"
  1-D Lookup Table3/1 -> Divide2/3  "r"
  Math Function3/1 -> Divide2/1, Sum1/1  "rd2"
  1-D Lookup Table2/1 -> Math Function3/1  "r"
  Sqrt/1 -> Divide1/2
  Divide1/1 -> MATLAB Function/2(vel), Sigmoid/1(u), Math Function2/1
  vel/1 -> To Workspace1/1, Divide1/1
  Constant2/1 -> Divide/2, Sqrt/1
  Demux/1 -> Atan2/2
  Sum/1 -> Math Function1/1, Divide/1, MATLAB Function/1(pos)  "acceleration"
  Demux/2 -> Atan2/1
  Atan2/1 -> 1-D Lookup Table2/1, 1-D Lookup Table3/1, 1-D Lookup Table1/1  "theta"
  Sum2/1 -> Torque1/1
  Input/1 -> Sum2/1
  Gain1/1 -> Sum2/2
  Sum1/1 -> Product/1, Scope/1, To Workspace3/1
  Product/1 -> Gain1/1
  Constant1/1 -> Sum/1
  MATLAB Function/1(Rot) -> Demux/1
  pos/1 -> Sum/2
  Sigmoid/1(y) -> Product/2
